simulink model "fxpdemo_fix2fixinh1"  (Simulink 7.6)
settings: Solver=FixedStepDiscrete  SolverMode=SingleTasking  StartTime=0.0  StopTime=0.9985  FixedStep=0.001  RelTol=1e-3  AbsTol=1e-6
libraries: simulink x1
Description:
  | Fixed-Point to Fixed-Point Inherited Conversion
  | 
  | Because of Simulink(R) ability to propagate data types throughout a block diagram,
  | fixed-point utility modeling can be templatized for multiple use scenarios.  The data
  | type inheritance capability can be given additional information through the use of
  | various relative-type specifications.  The FixPt To FixPt Inherited block provides a way
  | to specify that "this signal should have the same fixed-point data type as that signal"
  | by wiring it up to the signals of interest.
settings Model: MinMaxOverflowLogging=MinMaxAndOverflow  Creator=The MathWorks Inc.  CovMetricSettings=d  ExtModeTrigMode=oneshot  ExtModeArmWhenConnect=off  ExtModeAutoUpdateStatusClock=off
settings DataIOCC: LimitDataPoints=off  SignalLoggingName=sigsOut
settings OptimizationCC: BooleanDataType=off  InitFltsAndDblsToZero=on  EfficientMapNaN2IntZero=off
settings DebuggingCC: SaveWithParameterizedLinksMsg=none  SignalResolutionControl=TryResolveAllWithWarning  SolverPrmCheckMsg=none  MultiTaskDSMMsg=warning  MultiTaskCondExecSysMsg=none  IntegerOverflowMsg=none  ParameterDowncastMsg=warning  ParameterOverflowMsg=warning  ParameterPrecisionLossMsg=none  StrictBusMsg=None
settings HardwareCC: TargetUnknown=on
settings RTWCC: IncludeERTFirstTime=on
settings GRTTargetCC: TargetFcnLib=ansi_tfl_tmw.mat

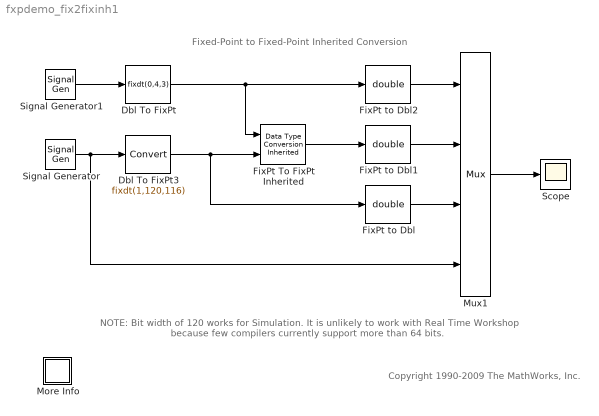
== system fxpdemo_fix2fixinh1 ==
  note: NOTE: Bit width of 120 works for Simulation.  It is unlikely to work with
      | Real Time Workshop because few compilers currently support more than 64 bits.
  note: Copyright 1990-2009 The MathWorks, Inc.
  note: Fixed-Point to Fixed-Point Inherited Conversion
  Dbl To FixPt : DataTypeConversion  OutDataTypeStr=fixdt(0,4,3)  RndMeth=Nearest  SaturateOnIntegerOverflow=on
  Dbl To FixPt3 : DataTypeConversion  OutDataTypeStr=fixdt(1,120,116)  SaturateOnIntegerOverflow=on
  FixPt To FixPt Inherited : simulink/Signal Attributes/Data Type Conversion Inherited  SystemSampleTime=-1  ConvertRealWorld=Real World Value  RndMeth=Nearest  DoSatur=on
  FixPt to Dbl : DataTypeConversion  OutDataTypeStr=double
  FixPt to Dbl1 : DataTypeConversion  OutDataTypeStr=double
  FixPt to Dbl2 : DataTypeConversion  OutDataTypeStr=double
  More Info : Subsystem
      settings: OpenFcn=showdemo(bdroot(gcs))
      mask Display: disp('?')
  Mux1 : Mux
  Scope : Scope
      settings: TickLabels=on
  Signal Generator : SignalGenerator  WaveForm=sawtooth  Amplitude=5
  Signal Generator1 : SignalGenerator  Frequency=10
  wires:
  Signal Generator1/1 -> Dbl To FixPt/1
  Dbl To FixPt/1 -> FixPt To FixPt Inherited/1, FixPt to Dbl2/1
  Dbl To FixPt3/1 -> FixPt To FixPt Inherited/2, FixPt to Dbl/1
  Signal Generator/1 -> Dbl To FixPt3/1, Mux1/4
  FixPt To FixPt Inherited/1 -> FixPt to Dbl1/1
  FixPt to Dbl1/1 -> Mux1/2
  FixPt to Dbl2/1 -> Mux1/1
  FixPt to Dbl/1 -> Mux1/3
  Mux1/1 -> Scope/1

== system fxpdemo_fix2fixinh1/More Info ==
